simulink model "H8_new_series_switching_upcoming_conference"  (R2018a)
settings: Solver=ode45  StartTime=0.0  StopTime=.02  RelTol=1e-3  EnableMultiTasking=on
libraries: powerlib x52, powerlib_extras x8, powerlib_meascontrol x6
settings Model: Creator=Personal  LastModifiedBy=HP
settings DataIOCC: LimitDataPoints=on  SaveFormat=Array
settings OptimizationCC: LifeSpan=inf
settings DebuggingCC: SolverPrmCheckMsg=warning  SFUnexpectedBacktrackingDiag=warning  SFNoUnconditionalDefaultTransitionDiag=warning  SFExecutionAtInitializationDiag=none
settings HardwareCC: ProdBitPerPointer=32  ProdBitPerSizeT=32  ProdBitPerPtrDiffT=32  ProdLargestAtomicFloat=None  ProdIntDivRoundTo=Undefined  ProdEndianess=Unspecified  ProdWordSize=32  ProdHWDeviceType=32-bit Generic
settings ModelReferenceCC: PropagateSignalLabelsOutOfModel=off
settings CodeAppCC: StateflowObjectComments=on
settings GRTTargetCC: TargetLangStandard=C89/C90 (ANSI)  GeneratePreprocessorConditionals=Disable all
settings ConfigComp: CovMetricSettings=dw  CovHtmlReporting=on  CovSaveCumulativeToWorkspaceVar=on  CovSaveSingleToWorkspaceVar=on  CovExternalEMLEnable=off  CovSFcnEnable=off
settings SimscapeCC: SimscapeNormalizeSystem=off

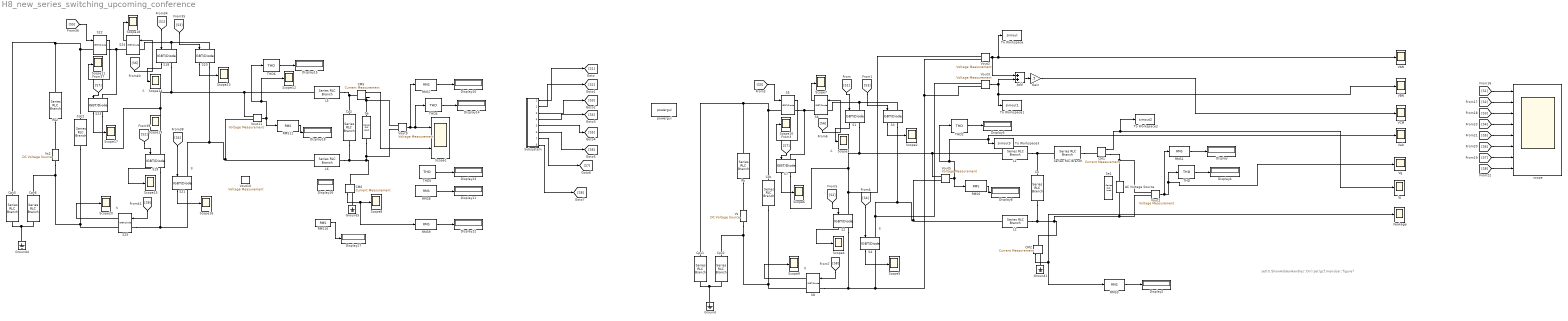
== system H8_new_series_switching_upcoming_conference ==
  note: set(0,'ShowHiddenHandles','On');set(gcf,'menubar','figure')
  note: A
  note: N
  note: B
  note: N
  note: A
  note: B
  AC Voltage Source : powerlib/Electrical Sources/AC Voltage Source  Amplitude=220  Phase=0  Frequency=50  SampleTime=0  Measurements=None  BusType=swing  Pref=10e3  Qref=0  Qmin=-inf  Qmax=+inf
  Add : Sum
  CM{1..2,5..6} (4 alike) : powerlib/Measurements/Current Measurement  PhasorSimulation=off  OutputType=Complex  PSBequivalent=0
  Cdc : powerlib/Elements/Series RLC Branch  LConnTagsString=__new0  RConnTagsString=__new0  BranchType=C  Resistance=1  Inductance=3e-3  SetiL0=off  InitialCurrent=0  Capacitance=940e-6  Setx0=off  InitialVoltage=0  Measurements=None
  Cdc2 : powerlib/Elements/Series RLC Branch  LConnTagsString=__new0  RConnTagsString=__new0  BranchType=C  Resistance=1  Inductance=3e-3  SetiL0=off  InitialCurrent=0  Capacitance=940e-6  Setx0=off  InitialVoltage=0  Measurements=None
  Co : powerlib/Elements/Series RLC Branch  LConnTagsString=__new0  RConnTagsString=__new0  BranchType=C  Resistance=1  Inductance=3e-3  SetiL0=off  InitialCurrent=0  Capacitance=2.2e-6  Setx0=off  InitialVoltage=0  Measurements=None
  Co2 : powerlib/Elements/Series RLC Branch  LConnTagsString=__new0  RConnTagsString=__new0  BranchType=C  Resistance=1  Inductance=3e-3  SetiL0=off  InitialCurrent=0  Capacitance=2.2e-6  Setx0=off  InitialVoltage=0  Measurements=None
  Cpv{1..2,5..6} (4 alike) : powerlib/Elements/Series RLC Branch  LConnTagsString=__new0  RConnTagsString=__new0  BranchType=C  Resistance=1  Inductance=3e-3  SetiL0=off  InitialCurrent=0  Capacitance=75e-9  Setx0=off  InitialVoltage=0  Measurements=None
  Display{,2,4..5,8,10..18} (14 alike) : Display
  Gain : Gain  Gain=.5
  Ground{,1,4..5} (4 alike) : powerlib/Elements/Ground  LConnTagsString=a
  Ig : Scope
  Ileakage : Scope
  L{1..2,5..6} (4 alike) : powerlib/Elements/Series RLC Branch  LConnTagsString=__new0  RConnTagsString=__new0  BranchType=L  Resistance=1  Inductance=3e-3  SetiL0=off  InitialCurrent=0  Capacitance=1e-6  Setx0=off  InitialVoltage=0  Measurements=None
  RMS{1,3,6..11} (8 alike) : powerlib_extras/Measurements/RMS  f1=50
  Rs : powerlib/Elements/Series RLC Branch  LConnTagsString=__new0  RConnTagsString=__new0  BranchType=R  Resistance=1  Inductance=3e-3  SetiL0=off  InitialCurrent=0  Capacitance=1e-6  Setx0=off  InitialVoltage=0  Measurements=None
  Rs2 : powerlib/Elements/Series RLC Branch  LConnTagsString=__new0  RConnTagsString=__new0  BranchType=R  Resistance=1  Inductance=3e-3  SetiL0=off  InitialCurrent=0  Capacitance=1e-6  Setx0=off  InitialVoltage=0  Measurements=None
  S{1..8,18..25} (16 alike) : powerlib/Power Electronics/IGBT//Diode  Ron=1e-3  Rs=1e5  Cs=inf  Measurements=on
  Scope1 : Scope  NumInputPorts=2
  Scope{2..20} (19 alike) : Scope
  Se : powerlib/Elements/Series RLC Load  LConnTagsString=a  RConnTagsString=__new0  NominalVoltage=230  NominalFrequency=50  ActivePower=1000  InductivePower=0  CapacitivePower=0  Setx0=off  InitialVoltage=0  SetiL0=off  InitialCurrent=0  Measurements=None  LoadType=constant Z
  Se1 : powerlib/Elements/Series RLC Load  LConnTagsString=a  RConnTagsString=__new0  NominalVoltage=230  NominalFrequency=50  ActivePower=1000  InductivePower=0  CapacitivePower=0  Setx0=off  InitialVoltage=0  SetiL0=off  InitialCurrent=0  Measurements=None  LoadType=constant Z
  Series RLC Branch : powerlib/Elements/Series RLC Branch  LConnTagsString=__new0  RConnTagsString=__new0  BranchType=R  Resistance=15  Inductance=1e-3  SetiL0=off  InitialCurrent=0  Capacitance=0  Setx0=off  InitialVoltage=0  Measurements=None
  Subsystem : Subsystem
  THD : powerlib_meascontrol/Measurements/THD  Freq=50  Ts=0
  THD2 : powerlib_meascontrol/Measurements/THD  Freq=60  Ts=0
  THD4 : powerlib_meascontrol/Measurements/THD  Freq=50  Ts=0
  THD5 : powerlib_meascontrol/Measurements/THD  Freq=50  Ts=0
  THD6 : powerlib_meascontrol/Measurements/THD  Freq=60  Ts=0
  To Workspace : ToWorkspace  VariableName=simout  SaveFormat=Timeseries  SampleTime=-1
  To Workspace1 : ToWorkspace  VariableName=simout1  SaveFormat=Timeseries  SampleTime=-1
  To Workspace2 : ToWorkspace  VariableName=simout2  SaveFormat=Timeseries  SampleTime=-1
  To Workspace3 : ToWorkspace  VariableName=simout3  SaveFormat=Timeseries  SampleTime=-1
  VAN : Scope
  VBN : Scope
  VCM : Scope
  Vab : Scope
  Vg : Scope
  Vout{1..3,5,9..11} (7 alike) : powerlib/Measurements/Voltage Measurement  PhasorSimulation=off  OutputType=Complex  PSBequivalent=0
  Vs : powerlib/Electrical Sources/DC Voltage Source  Amplitude=400  Measurements=None
  Vs2 : powerlib/Electrical Sources/DC Voltage Source  Amplitude=330  Measurements=None
  powergui : powerlib/powergui  Priority=1  SimulationMode=Continuous  SampleTime=50e-6  frequency=60  Iterations=50  frequencyindice=0  Pbase=100e6  ErrMax=1e-4  UnitsV=kV  UnitsW=MW  buscounter=0  FunctionMessages=off  echomessages=off  EnableUseOfTLC=off  CurrentSourceSwitches=off  DisableSnubberDevices=off  DisableRonSwitches=off  DisableVfSwitches=off  DisplayEquations=off  SolverType=Tustin/Backward Euler (TBE)  Interpol=off  ExternalGateDelay=off  methode=off  Ts=100  x0status=blocks  SPID=on  SwTol=0  HookPort=off  RestoreLinks=warning  ResistiveCurrentMeasurement=off  Frange=[0:2:500]  Ylog=off  Xlog=on  ShowGrid=off  save=off  variable=ZData  structure=Vg  ZoomFFT=off  StartTime=0  cycles=2  DisplayStyle=1  fundamental=50  FreqAxis=off  MaxFrequency=10000  frequencyindicesteady=1  RmsSteady=1  display=off
  scope : Scope  NumInputPorts=8
  wires:
  Subsystem/1(Out1) -> [S1]
  Subsystem/2(Out2) -> [S2]
  Subsystem/3(Out3) -> [S3]
  Subsystem/4(Out4) -> [S4]
  Subsystem/5(Out5) -> [S5]
  [S1] -> S1/1
  [S3] -> S3/1
  Vout1/1 -> RMS1/1, THD/1, Vg/1
  THD/1 -> Display4/1
  [S4] -> S4/1
  [S2] -> S2/1
  RMS3/1 -> Display2/1
  CM2/1 -> RMS3/1, Ileakage/1
  RMS1/1 -> Display/1
  THD2/1 -> Display5/1
  Vout5/1 -> To Workspace3/1, Vab/1, THD2/1, RMS6/1
  RMS6/1 -> Display8/1
  S3/1 -> Scope2/1
  S1/1 -> Scope3/1
  S2/1 -> Scope4/1
  S4/1 -> Scope5/1
  S5/1 -> Scope10/1
  [S5] -> S5/1
  S7/1 -> Scope6/1
  [S7] -> S7/1
  S6/1 -> Scope7/1
  [S6] -> S6/1
  Subsystem/6(Out6) -> [S6]
  Subsystem/7(Out7) -> [S7]
  [S8] -> S8/1
  S8/1 -> Scope9/1
  Subsystem/8(Out8) -> [S8]
  Vout2/1 -> Add/1, To Workspace/1, VAN/1
  Vout3/1 -> Add/2, To Workspace1/1, VBN/1
  CM1/1 -> To Workspace2/1, Ig/1
  Gain/1 -> VCM/1
  Add/1 -> Gain/1
  [S1] -> scope/1
  [S2] -> scope/2
  [S3] -> scope/3
  [S4] -> scope/4
  [S5] -> scope/5
  [S6] -> scope/6
  [S8] -> scope/8
  [S7] -> scope/7
  ? -> Display16/1
  Vout9/1 -> RMS7/1, THD4/1, Scope1/1
  [S5] -> S22/1
  THD6/1 -> Display15/1
  S25/1 -> Scope20/1
  [S1] -> S18/1
  THD4/1 -> Display14/1
  [S3] -> S20/1
  S24/1 -> Scope18/1
  [S6] -> S24/1
  [S7] -> S23/1
  S20/1 -> Scope13/1
  Vout11/1 -> Scope12/1, THD6/1, RMS11/1
  RMS11/1 -> Display18/1
  [S8] -> S25/1
  S18/1 -> Scope14/1
  RMS8/1 -> Display11/1
  S22/1 -> Scope11/1
  RMS7/1 -> Display10/1
  RMS9/1 -> Display12/1
  S23/1 -> Scope17/1
  [S2] -> S19/1
  S21/1 -> Scope16/1
  [S4] -> S21/1
  RMS10/1 -> Display17/1
  THD5/1 -> Display13/1
  S19/1 -> Scope15/1
  CM5/1 -> Scope1/2
  CM6/1 -> RMS9/1, Scope8/1
  connections:
  Cdc/LConn1 -- Rs/RConn1 -- Cpv1/LConn1 -- S5/LConn1
  S1/RConn1 -- Vout2/LConn1 -- S2/LConn1 -- S7/RConn1 -- Vout5/LConn1 -- L1/LConn1
  Ground/LConn1 -- Cpv2/RConn1 -- Cpv1/RConn1
  Vout5/LConn2 -- L2/LConn1 -- Vout3/LConn1 -- S4/LConn1 -- S3/RConn1
  Ground1/LConn1 -- CM2/RConn1
  Rs/LConn1 -- Vs/RConn1
  Vs/LConn1 -- S8/RConn1 -- Cdc/RConn1 -- Cpv2/LConn1
  Series RLC Branch/RConn1 -- CM1/LConn1
  L2/RConn1 -- Co/RConn1 -- Vout1/LConn2 -- AC Voltage Source/LConn1 -- CM2/LConn1
  CM1/RConn1 -- Vout1/LConn1 -- AC Voltage Source/RConn1
  S5/RConn1 -- S6/RConn1 -- S7/LConn1
  S3/LConn1 -- S1/LConn1 -- S6/LConn1
  S8/LConn1 -- S2/RConn1 -- Vout3/LConn2 -- Vout2/LConn2 -- S4/RConn1
  Co/LConn1 -- Series RLC Branch/LConn1 -- L1/RConn1
  S23/LConn1 -- S22/RConn1 -- S24/RConn1
  CM6/LConn1 -- Vout9/LConn2 -- Se/RConn1 -- L6/RConn1 -- Co2/RConn1
  S20/RConn1 -- Vout11/LConn2 -- L6/LConn1 -- S21/LConn1
  Co2/LConn1 -- L5/RConn1 -- CM5/LConn1
  S19/LConn1 -- S18/RConn1 -- Vout11/LConn1 -- L5/LConn1 -- S23/RConn1
  Cpv6/LConn1 -- Vs2/LConn1 -- Cdc2/RConn1 -- S25/RConn1
  S22/LConn1 -- Cdc2/LConn1 -- Rs2/RConn1 -- Cpv5/LConn1
  S21/RConn1 -- S25/LConn1 -- S19/RConn1
  Se/LConn1 -- CM5/RConn1 -- Vout9/LConn1
  S24/LConn1 -- S20/LConn1 -- S18/LConn1
  Cpv5/RConn1 -- Ground4/LConn1 -- Cpv6/RConn1
  Rs2/LConn1 -- Vs2/RConn1
  Ground5/LConn1 -- CM6/RConn1

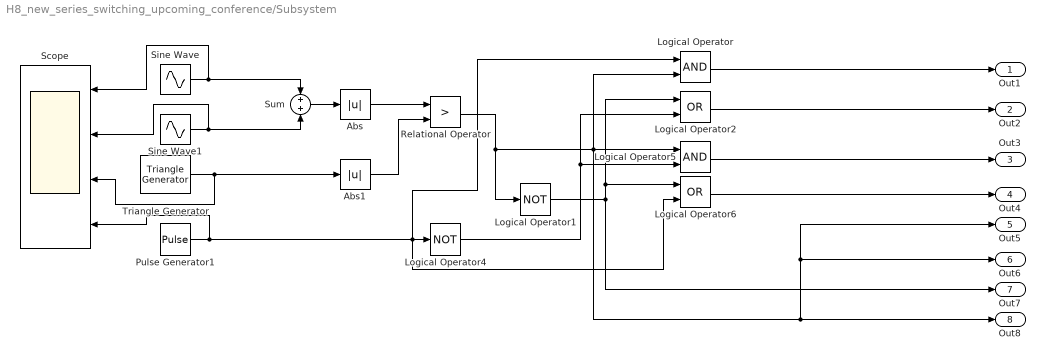
== system H8_new_series_switching_upcoming_conference/Subsystem ==
  Abs : Abs
  Abs1 : Abs
  Logical Operator : Logic  AllPortsSameDT=off  OutDataTypeStr=boolean
  Logical Operator1 : Logic  Operator=NOT  AllPortsSameDT=off  OutDataTypeStr=boolean
  Logical Operator2 : Logic  Operator=OR  AllPortsSameDT=off  OutDataTypeStr=boolean
  Logical Operator4 : Logic  Operator=NOT  AllPortsSameDT=off  OutDataTypeStr=boolean
  Logical Operator5 : Logic  AllPortsSameDT=off  OutDataTypeStr=boolean
  Logical Operator6 : Logic  Operator=OR  AllPortsSameDT=off  OutDataTypeStr=boolean
  Pulse Generator1 : DiscretePulseGenerator  PulseType=Time based  Period=.02  PulseWidth=50
  Relational Operator : RelationalOperator  Operator=>  OutDataTypeStr=boolean  RndMeth=Nearest
  Scope : Scope  NumInputPorts=4
  Sine Wave : Sin  Frequency=2*pi*50  SampleTime=0
  Sine Wave1 : Sin  Amplitude=.003  Frequency=2*pi*3*50  Phase=pi  SampleTime=0
  Sum : Sum
  Triangle Generator : powerlib_meascontrol/Pulse & Signal Generators/Triangle Generator  Freq=8e3  Phase=90  Ts=0
  Out1 : Outport
  Out2 : Outport  Port=2
  Out3 : Outport  Port=3
  Out4 : Outport  Port=4
  Out5 : Outport  Port=5
  Out6 : Outport  Port=6
  Out7 : Outport  Port=7
  Out8 : Outport  Port=8
  wires:
  Relational Operator/1 -> Logical Operator1/1, Out6/1, Out5/1, Out8/1, Logical Operator5/1, Logical Operator/2
  Abs1/1 -> Relational Operator/2
  Abs/1 -> Relational Operator/1
  Sine Wave/1 -> Scope/1, Sum/1
  Sum/1 -> Abs/1
  Pulse Generator1/1 -> Scope/4, Logical Operator/1, Logical Operator6/2, Logical Operator4/1
  Logical Operator4/1 -> Logical Operator2/2, Logical Operator5/2
  Logical Operator1/1 -> Logical Operator6/1, Logical Operator2/1, Out7/1
  Sine Wave1/1 -> Scope/2, Sum/2
  Logical Operator/1 -> Out1/1
  Logical Operator5/1 -> Out3/1
  Logical Operator6/1 -> Out4/1
  Logical Operator2/1 -> Out2/1
  Triangle Generator/1 -> Scope/3, Abs1/1
